simulink model "active_vehicle_controller_functions"  (R2020a)
settings: Solver=ode4  StartTime=0.0  StopTime=inf  FixedStep=1e-3  RelTol=1e-3
InitFcn:
  | clear mex
undefined symbols (not defined in the file or in its folder): DiscIntNeverNeededParam, vicrt_initcallback, vicrt_initmexcallback, vicrt_inputfile, vicrt_simulationmanager
libraries: simulink x1
(part 2 of 6)

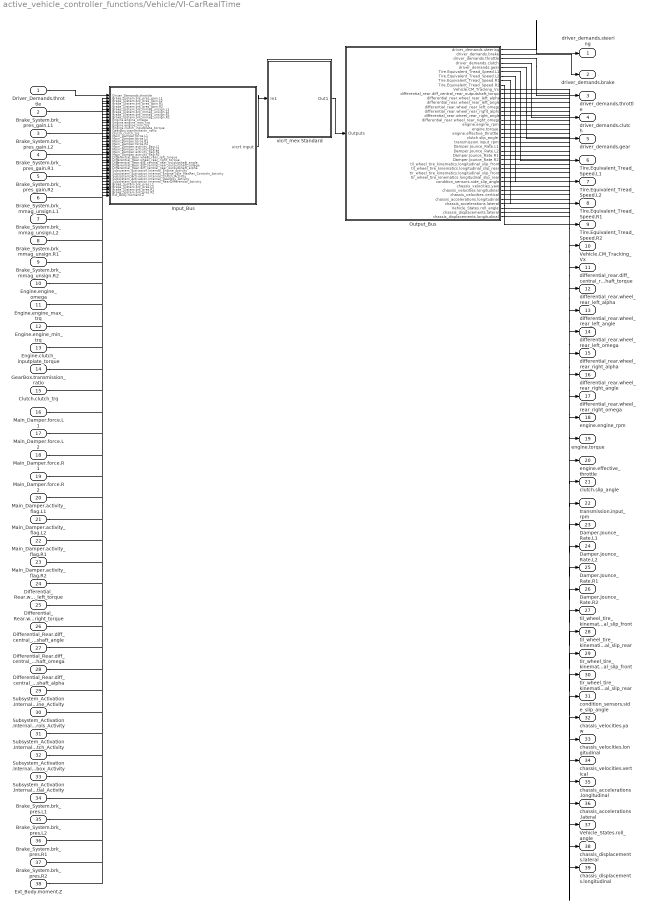
== system active_vehicle_controller_functions/Vehicle/VI-CarRealTime ==
  Driver_Demands.throttle : Inport
  Brake_System.brk_pres_gain.L1 : Inport  Port=2
  Brake_System.brk_pres_gain.L2 : Inport  Port=3
  Brake_System.brk_pres_gain.R1 : Inport  Port=4
  Brake_System.brk_pres_gain.R2 : Inport  Port=5
  Brake_System.brk_mmag_unsign.L1 : Inport  Port=6
  Brake_System.brk_mmag_unsign.L2 : Inport  Port=7
  Brake_System.brk_mmag_unsign.R1 : Inport  Port=8
  Brake_System.brk_mmag_unsign.R2 : Inport  Port=9
  Engine.engine_omega : Inport  Port=10
  Engine.engine_max_trq : Inport  Port=11
  Engine.engine_min_trq : Inport  Port=12
  Engine.clutch_inputplate_torque : Inport  Port=13
  GearBox.transmission_ratio : Inport  Port=14
  Clutch.clutch_trq : Inport  Port=15
  Main_Damper.force.L1 : Inport  Port=16
  Main_Damper.force.L2 : Inport  Port=17
  Main_Damper.force.R1 : Inport  Port=18
  Main_Damper.force.R2 : Inport  Port=19
  Main_Damper.activity_flag.L1 : Inport  Port=20
  Main_Damper.activity_flag.L2 : Inport  Port=21
  Main_Damper.activity_flag.R1 : Inport  Port=22
  Main_Damper.activity_flag.R2 : Inport  Port=23
  Differential_Rear.wheel_rear_left_torque : Inport  Port=24
  Differential_Rear.wheel_rear_right_torque : Inport  Port=25
  Differential_Rear.diff_central_rear_outputshaft_angle : Inport  Port=26
  Differential_Rear.diff_central_rear_outputshaft_omega : Inport  Port=27
  Differential_Rear.diff_central_rear_outputshaft_alpha : Inport  Port=28
  Subsystem_Activation.Internal_Engine_Activity : Inport  Port=29
  Subsystem_Activation.Internal_Engine_Idle_MaxRev_Controls_Activity : Inport  Port=30
  Subsystem_Activation.Internal_Clutch_Activity : Inport  Port=31
  Subsystem_Activation.Internal_Gearbox_Activity : Inport  Port=32
  Subsystem_Activation.Internal_RearDifferential_Activity : Inport  Port=33
  Brake_System.brk_pres.L1 : Inport  Port=34
  Brake_System.brk_pres.L2 : Inport  Port=35
  Brake_System.brk_pres.R1 : Inport  Port=36
  Brake_System.brk_pres.R2 : Inport  Port=37
  Ext_Body.moment.Z : Inport  Port=38
  Input_Bus : Subsystem  LoadFcn=vicrt_initcallback(gcb)
      settings: CopyFcn=vicrt_initcallback(gcb)
  Output_Bus : Subsystem  Description=Outputs
      settings: CopyFcn=set_param(gcb, 'LinkStatus', 'none')
  vicrt_mex Standard : Subsystem  mask{vicrt_inputfile=vicrt_inputfile, vicrt_outprefix='', intStep=0.001, AniFlag=on, inpPortDim=389, outPortDim=1374, NoDirectFeedthrough=on}
      mask prompts: vicrt_inputfile "VI-CarRealtime input file"; vicrt_outprefix "VI-CarRealTime output prefix"; intStep "Integration step"; AniFlag "live animation"; inpPortDim "input port dimension"; outPortDim "output port dimension"; NoDirectFeedthrough "Direct Feedthrough Off"
      mask init:
      | custDriv=[1,1,1];
      settings: CopyFcn=set_param(gcb, 'LinkStatus', 'none')
  driver_demands.steering : Outport  VectorParamsAs1DForOutWhenUnconnected=off
  driver_demands.brake : Outport  Port=2  VectorParamsAs1DForOutWhenUnconnected=off
  driver_demands.throttle : Outport  Port=3  VectorParamsAs1DForOutWhenUnconnected=off
  driver_demands.clutch : Outport  Port=4  VectorParamsAs1DForOutWhenUnconnected=off
  driver_demands.gear : Outport  Port=5  VectorParamsAs1DForOutWhenUnconnected=off
  Tire.Equivalent_Tread_Speed.L1 : Outport  Port=6  VectorParamsAs1DForOutWhenUnconnected=off
  Tire.Equivalent_Tread_Speed.L2 : Outport  Port=7  VectorParamsAs1DForOutWhenUnconnected=off
  Tire.Equivalent_Tread_Speed.R1 : Outport  Port=8  VectorParamsAs1DForOutWhenUnconnected=off
  Tire.Equivalent_Tread_Speed.R2 : Outport  Port=9  VectorParamsAs1DForOutWhenUnconnected=off
  Vehicle.CM_Tracking_Vx : Outport  Port=10  VectorParamsAs1DForOutWhenUnconnected=off
  differential_rear.diff_central_rear_outputshaft_torque : Outport  Port=11  VectorParamsAs1DForOutWhenUnconnected=off
  differential_rear.wheel_rear_left_alpha : Outport  Port=12  VectorParamsAs1DForOutWhenUnconnected=off
  differential_rear.wheel_rear_left_angle : Outport  Port=13  VectorParamsAs1DForOutWhenUnconnected=off
  differential_rear.wheel_rear_left_omega : Outport  Port=14  VectorParamsAs1DForOutWhenUnconnected=off
  differential_rear.wheel_rear_right_alpha : Outport  Port=15  VectorParamsAs1DForOutWhenUnconnected=off
  differential_rear.wheel_rear_right_angle : Outport  Port=16  VectorParamsAs1DForOutWhenUnconnected=off
  differential_rear.wheel_rear_right_omega : Outport  Port=17  VectorParamsAs1DForOutWhenUnconnected=off
  engine.engine_rpm : Outport  Port=18  VectorParamsAs1DForOutWhenUnconnected=off
  engine.torque : Outport  Port=19  VectorParamsAs1DForOutWhenUnconnected=off
  engine.effective_throttle : Outport  Port=20  VectorParamsAs1DForOutWhenUnconnected=off
  clutch.slip_angle : Outport  Port=21  VectorParamsAs1DForOutWhenUnconnected=off
  transmission.input_rpm : Outport  Port=22  VectorParamsAs1DForOutWhenUnconnected=off
  Damper.Jounce_Rate.L1 : Outport  Port=23  VectorParamsAs1DForOutWhenUnconnected=off
  Damper.Jounce_Rate.L2 : Outport  Port=24  VectorParamsAs1DForOutWhenUnconnected=off
  Damper.Jounce_Rate.R1 : Outport  Port=25  VectorParamsAs1DForOutWhenUnconnected=off
  Damper.Jounce_Rate.R2 : Outport  Port=26  VectorParamsAs1DForOutWhenUnconnected=off
  til_wheel_tire_kinematics.longitudinal_slip_front : Outport  Port=27  VectorParamsAs1DForOutWhenUnconnected=off
  til_wheel_tire_kinematics.longitudinal_slip_rear : Outport  Port=28  VectorParamsAs1DForOutWhenUnconnected=off
  tir_wheel_tire_kinematics.longitudinal_slip_front : Outport  Port=29  VectorParamsAs1DForOutWhenUnconnected=off
  tir_wheel_tire_kinematics.longitudinal_slip_rear : Outport  Port=30  VectorParamsAs1DForOutWhenUnconnected=off
  condition_sensors.side_slip_angle : Outport  Port=31  VectorParamsAs1DForOutWhenUnconnected=off
  chassis_velocities.yaw : Outport  Port=32  VectorParamsAs1DForOutWhenUnconnected=off
  chassis_velocities.longitudinal : Outport  Port=33  VectorParamsAs1DForOutWhenUnconnected=off
  chassis_velocities.vertical : Outport  Port=34  VectorParamsAs1DForOutWhenUnconnected=off
  chassis_accelerations.longitudinal : Outport  Port=35  VectorParamsAs1DForOutWhenUnconnected=off
  chassis_accelerations.lateral : Outport  Port=36  VectorParamsAs1DForOutWhenUnconnected=off
  Vehicle_States.roll_angle : Outport  Port=37
  chassis_displacements.lateral : Outport  Port=38
  chassis_displacements.longitudinal : Outport  Port=39
  wires:
  vicrt_mex Standard/1(Out1) -> Output_Bus/1(Outputs)
  Input_Bus/1(vicrt input) -> vicrt_mex Standard/1(In1)
  Driver_Demands.throttle/1 -> Input_Bus/1(Driver_Demands.throttle)
  Brake_System.brk_pres_gain.L1/1 -> Input_Bus/2(Brake_System.brk_pres_gain.L1)
  Brake_System.brk_pres_gain.L2/1 -> Input_Bus/3(Brake_System.brk_pres_gain.L2)
  Brake_System.brk_pres_gain.R1/1 -> Input_Bus/4(Brake_System.brk_pres_gain.R1)
  Brake_System.brk_pres_gain.R2/1 -> Input_Bus/5(Brake_System.brk_pres_gain.R2)
  Brake_System.brk_mmag_unsign.L1/1 -> Input_Bus/6(Brake_System.brk_mmag_unsign.L1)
  Brake_System.brk_mmag_unsign.L2/1 -> Input_Bus/7(Brake_System.brk_mmag_unsign.L2)
  Brake_System.brk_mmag_unsign.R1/1 -> Input_Bus/8(Brake_System.brk_mmag_unsign.R1)
  Brake_System.brk_mmag_unsign.R2/1 -> Input_Bus/9(Brake_System.brk_mmag_unsign.R2)
  Engine.engine_omega/1 -> Input_Bus/10(Engine.engine_omega)
  Engine.engine_max_trq/1 -> Input_Bus/11(Engine.engine_max_trq)
  Engine.engine_min_trq/1 -> Input_Bus/12(Engine.engine_min_trq)
  Engine.clutch_inputplate_torque/1 -> Input_Bus/13(Engine.clutch_inputplate_torque)
  GearBox.transmission_ratio/1 -> Input_Bus/14(GearBox.transmission_ratio)
  Clutch.clutch_trq/1 -> Input_Bus/15(Clutch.clutch_trq)
  Main_Damper.force.L1/1 -> Input_Bus/16(Main_Damper.force.L1)
  Main_Damper.force.L2/1 -> Input_Bus/17(Main_Damper.force.L2)
  Main_Damper.force.R1/1 -> Input_Bus/18(Main_Damper.force.R1)
  Main_Damper.force.R2/1 -> Input_Bus/19(Main_Damper.force.R2)
  Main_Damper.activity_flag.L1/1 -> Input_Bus/20(Main_Damper.activity_flag.L1)
  Main_Damper.activity_flag.L2/1 -> Input_Bus/21(Main_Damper.activity_flag.L2)
  Main_Damper.activity_flag.R1/1 -> Input_Bus/22(Main_Damper.activity_flag.R1)
  Main_Damper.activity_flag.R2/1 -> Input_Bus/23(Main_Damper.activity_flag.R2)
  Differential_Rear.wheel_rear_left_torque/1 -> Input_Bus/24(Differential_Rear.wheel_rear_left_torque)
  Differential_Rear.wheel_rear_right_torque/1 -> Input_Bus/25(Differential_Rear.wheel_rear_right_torque)
  Differential_Rear.diff_central_rear_outputshaft_angle/1 -> Input_Bus/26(Differential_Rear.diff_central_rear_outputshaft_angle)
  Differential_Rear.diff_central_rear_outputshaft_omega/1 -> Input_Bus/27(Differential_Rear.diff_central_rear_outputshaft_omega)
  Differential_Rear.diff_central_rear_outputshaft_alpha/1 -> Input_Bus/28(Differential_Rear.diff_central_rear_outputshaft_alpha)
  Subsystem_Activation.Internal_Engine_Activity/1 -> Input_Bus/29(Subsystem_Activation.Internal_Engine_Activity)
  Subsystem_Activation.Internal_Engine_Idle_MaxRev_Controls_Activity/1 -> Input_Bus/30(Subsystem_Activation.Internal_Engine_Idle_MaxRev_Controls_Activity)
  Subsystem_Activation.Internal_Clutch_Activity/1 -> Input_Bus/31(Subsystem_Activation.Internal_Clutch_Activity)
  Subsystem_Activation.Internal_Gearbox_Activity/1 -> Input_Bus/32(Subsystem_Activation.Internal_Gearbox_Activity)
  Subsystem_Activation.Internal_RearDifferential_Activity/1 -> Input_Bus/33(Subsystem_Activation.Internal_RearDifferential_Activity)
  Brake_System.brk_pres.L1/1 -> Input_Bus/34(Brake_System.brk_pres.L1)
  Brake_System.brk_pres.L2/1 -> Input_Bus/35(Brake_System.brk_pres.L2)
  Brake_System.brk_pres.R1/1 -> Input_Bus/36(Brake_System.brk_pres.R1)
  Brake_System.brk_pres.R2/1 -> Input_Bus/37(Brake_System.brk_pres.R2)
  Ext_Body.moment.Z/1 -> Input_Bus/38(Ext_Body.moment.Z)
  Output_Bus/1(driver_demands.steering) -> driver_demands.steering/1
  Output_Bus/2(driver_demands.brake) -> driver_demands.brake/1
  Output_Bus/3(driver_demands.throttle) -> driver_demands.throttle/1
  Output_Bus/4(driver_demands.clutch) -> driver_demands.clutch/1
  Output_Bus/5(driver_demands.gear) -> driver_demands.gear/1
  Output_Bus/6(Tire.Equivalent_Tread_Speed.L1) -> Tire.Equivalent_Tread_Speed.L1/1
  Output_Bus/7(Tire.Equivalent_Tread_Speed.L2) -> Tire.Equivalent_Tread_Speed.L2/1
  Output_Bus/8(Tire.Equivalent_Tread_Speed.R1) -> Tire.Equivalent_Tread_Speed.R1/1
  Output_Bus/9(Tire.Equivalent_Tread_Speed.R2) -> Tire.Equivalent_Tread_Speed.R2/1
  Output_Bus/10(Vehicle.CM_Tracking_Vx) -> Vehicle.CM_Tracking_Vx/1
  Output_Bus/11(differential_rear.diff_central_rear_outputshaft_torque) -> differential_rear.diff_central_rear_outputshaft_torque/1
  Output_Bus/12(differential_rear.wheel_rear_left_alpha) -> differential_rear.wheel_rear_left_alpha/1
  Output_Bus/13(differential_rear.wheel_rear_left_angle) -> differential_rear.wheel_rear_left_angle/1
  Output_Bus/14(differential_rear.wheel_rear_left_omega) -> differential_rear.wheel_rear_left_omega/1
  Output_Bus/15(differential_rear.wheel_rear_right_alpha) -> differential_rear.wheel_rear_right_alpha/1
  Output_Bus/16(differential_rear.wheel_rear_right_angle) -> differential_rear.wheel_rear_right_angle/1
  Output_Bus/17(differential_rear.wheel_rear_right_omega) -> differential_rear.wheel_rear_right_omega/1
  Output_Bus/18(engine.engine_rpm) -> engine.engine_rpm/1
  Output_Bus/19(engine.torque) -> engine.torque/1
  Output_Bus/20(engine.effective_throttle) -> engine.effective_throttle/1
  Output_Bus/21(clutch.slip_angle) -> clutch.slip_angle/1
  Output_Bus/22(transmission.input_rpm) -> transmission.input_rpm/1
  Output_Bus/23(Damper.Jounce_Rate.L1) -> Damper.Jounce_Rate.L1/1
  Output_Bus/24(Damper.Jounce_Rate.L2) -> Damper.Jounce_Rate.L2/1
  Output_Bus/25(Damper.Jounce_Rate.R1) -> Damper.Jounce_Rate.R1/1
  Output_Bus/26(Damper.Jounce_Rate.R2) -> Damper.Jounce_Rate.R2/1
  Output_Bus/27(til_wheel_tire_kinematics.longitudinal_slip_front) -> til_wheel_tire_kinematics.longitudinal_slip_front/1
  Output_Bus/28(til_wheel_tire_kinematics.longitudinal_slip_rear) -> til_wheel_tire_kinematics.longitudinal_slip_rear/1
  Output_Bus/29(tir_wheel_tire_kinematics.longitudinal_slip_front) -> tir_wheel_tire_kinematics.longitudinal_slip_front/1
  Output_Bus/30(tir_wheel_tire_kinematics.longitudinal_slip_rear) -> tir_wheel_tire_kinematics.longitudinal_slip_rear/1
  Output_Bus/31(condition_sensors.side_slip_angle) -> condition_sensors.side_slip_angle/1
  Output_Bus/32(chassis_velocities.yaw) -> chassis_velocities.yaw/1
  Output_Bus/33(chassis_velocities.longitudinal) -> chassis_velocities.longitudinal/1
  Output_Bus/34(chassis_velocities.vertical) -> chassis_velocities.vertical/1
  Output_Bus/35(chassis_accelerations.longitudinal) -> chassis_accelerations.longitudinal/1
  Output_Bus/36(chassis_accelerations.lateral) -> chassis_accelerations.lateral/1
  Output_Bus/37(Vehicle_States.roll_angle) -> Vehicle_States.roll_angle/1
  Output_Bus/38(chassis_displacements.lateral) -> chassis_displacements.lateral/1
  Output_Bus/39(chassis_displacements.longitudinal) -> chassis_displacements.longitudinal/1

== system active_vehicle_controller_functions/Driveline/Clutch/lag ==
  In1 : Inport
  Memory5 : Memory  InheritSampleTime=on
  Sum : Sum  Inputs=|++  OutDataTypeStr=Inherit: Same as first input
  "gain_1 " : Gain  Gain=1-exp(-2*pi*0.001)  OutDataTypeStr=Inherit: Same as input  ParamDataTypeStr=Inherit: Same as input
  gain_1 1 : Gain  Gain=exp(-2*pi*0.001)  OutDataTypeStr=Inherit: Same as input  ParamDataTypeStr=Inherit: Same as input
  Out1 : Outport  VectorParamsAs1DForOutWhenUnconnected=off
  wires:
  In1/1 -> "gain_1 "/1
  "gain_1 "/1 -> Sum/1
  Sum/1 -> Memory5/1, Out1/1
  Memory5/1 -> gain_1 1/1
  gain_1 1/1 -> Sum/2

== system active_vehicle_controller_functions/Driveline/Engine/Engine Maps ==
  RPM : Inport
  Throttle : Inport  Port=2
  0-throttle : Constant  Value=0
  Demux : Demux  Outputs=3
  Engine Torque : Lookup2D  RowIndex=|  ColumnIndex=[0,1]  Table="[0.0  0.0; -20.0  120.0;-42.0  270.0; -44.0  400.0;-46.0  490.0; -48.0  526.0;-50.0  620.0; -50.0  716.0;-50.0  808.0; -50.0  910.0; -50.0  950.0; -50.0  970.0;-50.0  936.0; -50.0  924.0; -52.0  910.0; -56.0  854.0; -60.0  740.0; -64.0  690.0; -68.0  650.0;]"
      | [0.0	
      | 500.0	
      | 1000.0	
      | 1500.0	
      | 2000.0	
      | 2500.0	
      | 3000.0	
      | 3500.0	
      | 4000.0	
      | 4500.0	
      | 5000.0	
      | 5500.0	
      | 6000.0	
      | 6250.0	
      | 6500.0	
      | 6750.0	
      | 7000.0	
      | 7500.0	
      | 8000.0]
  FullThrottle : Constant
  Memory1 : Memory
  Mux : Mux  Inputs=3
  Rpm control : Subsystem
  Saturation Dynamic : simulink/Discontinuities/Saturation Dynamic  OutMin=[]  OutMax=[]  OutDataTypeStr=Inherit: Same as second input  OutDataType=sfix(16)  OutScaling=2^-10  DoSatur=off
  Switch : Switch  Criteria=u2 > Threshold
  Zero : Constant  Value=[0,0,0]
  rpm2rad_sec : Gain  Gain=(60/2/pi)^-1  OutDataTypeStr=Inherit: Same as input  ParamDataTypeStr=Inherit: Same as input
  scale : Gain  Gain=0.01  OutDataTypeStr=Inherit: Same as input  ParamDataTypeStr=Inherit: Same as input
  MaxEngineTorque : Outport  VectorParamsAs1DForOutWhenUnconnected=off
  MinEngineTorque : Outport  Port=2  VectorParamsAs1DForOutWhenUnconnected=off
  EngineTorque : Outport  Port=3  VectorParamsAs1DForOutWhenUnconnected=off
  wires:
  Throttle/1 -> Rpm control/2(Throttle)
  scale/1 -> Mux/2
  FullThrottle/1 -> Mux/1
  Mux/1 -> Engine Torque/2
  RPM/1 -> Engine Torque/1, rpm2rad_sec/1
  Demux/1 -> MaxEngineTorque/1, Saturation Dynamic/1
  Demux/3 -> MinEngineTorque/1, Saturation Dynamic/3
  rpm2rad_sec/1 -> Rpm control/1(engine omega)
  0-throttle/1 -> Mux/3
  Rpm control/1(Throttle mod) -> scale/1
  Saturation Dynamic/1 -> EngineTorque/1
  Demux/2 -> Saturation Dynamic/2
  [InternalEngineActive] -> Switch/2
  Zero/1 -> Switch/1
  Switch/1 -> Demux/1
  Memory1/1 -> Switch/3
  Engine Torque/1 -> Memory1/1

== system active_vehicle_controller_functions/Driveline/Engine/ThrottleOff (from ESP) ==
  Constant : Constant
  Sum : Sum  Inputs=|+-  OutDataTypeStr=Inherit: Same as first input
  ThrottleOffGain1 : Gain  Gain=1-ThrottleOffScale  OutDataTypeStr=Inherit: Same as input  ParamDataTypeStr=Inherit: Same as input
  Transfer Fcn : TransferFcn  Denominator="[0.02  1]"
  ThrottleGain : Outport  VectorParamsAs1DForOutWhenUnconnected=off
  wires:
  ThrottleOffGain1/1 -> Transfer Fcn/1
  Constant/1 -> Sum/1
  Transfer Fcn/1 -> Sum/2
  [ThrottleOff] -> ThrottleOffGain1/1
  Sum/1 -> ThrottleGain/1

== system active_vehicle_controller_functions/Driveline/Rear Differential/Limited Slip Diff ==
  diff center front output shaft torque : Inport
  wheel front right omega : Inport  Port=2
  wheel front left omega : Inport  Port=3
  " " : Memory
  "   " : Memory
  "    " : Memory
  "       " : Memory
  "          " : Math  Operator=pow  SignedPower=on  SaturateOnIntegerOverflow=on
  AbsDeltaOmega : Abs
  AbsT : Abs
  C0 : Constant  Value=C0
  C1 : Gain  Gain=C1
  C2 : Gain  Gain=C2
  C3 : Constant  Value=C3
  C4 : Gain  Gain=-1
  DeltaTorqueL : Product  Inputs=**
  DeltaTorqueR : Product  Inputs=**
  Sign : Lookup  InputValues=[-1000 -100 -1 -0.5 0 .5 1 100 1000]  Table=[-1 -1 -1 0 0 0 1 1 1]
  Sum : Sum  Inputs=+-
  Sum3 : Sum  Inputs=+++  SaturateOnIntegerOverflow=on
  wheel front left torque : Outport  VectorParamsAs1DForOutWhenUnconnected=off
  wheel front right torque : Outport  Port=2  VectorParamsAs1DForOutWhenUnconnected=off
  wires:
  C0/1 -> Sum3/1
  C2/1 -> "          "/1
  "    "/1 -> DeltaTorqueL/2, DeltaTorqueR/2
  "       "/1 -> Sum3/3
  DeltaTorqueR/1 -> C4/1
  Sign/1 -> "    "/1
  C1/1 -> Sum3/2
  Sum3/1 -> DeltaTorqueR/1, DeltaTorqueL/1
  C4/1 -> wheel front right torque/1
  AbsT/1 -> "   "/1
  "          "/1 -> "       "/1
  AbsDeltaOmega/1 -> " "/1
  wheel front left omega/1 -> Sum/2
  "   "/1 -> C1/1
  diff center front output shaft torque/1 -> AbsT/1
  " "/1 -> C2/1
  DeltaTorqueL/1 -> wheel front left torque/1
  C3/1 -> "          "/2
  Sum/1 -> Sign/1, AbsDeltaOmega/1
  wheel front right omega/1 -> Sum/1

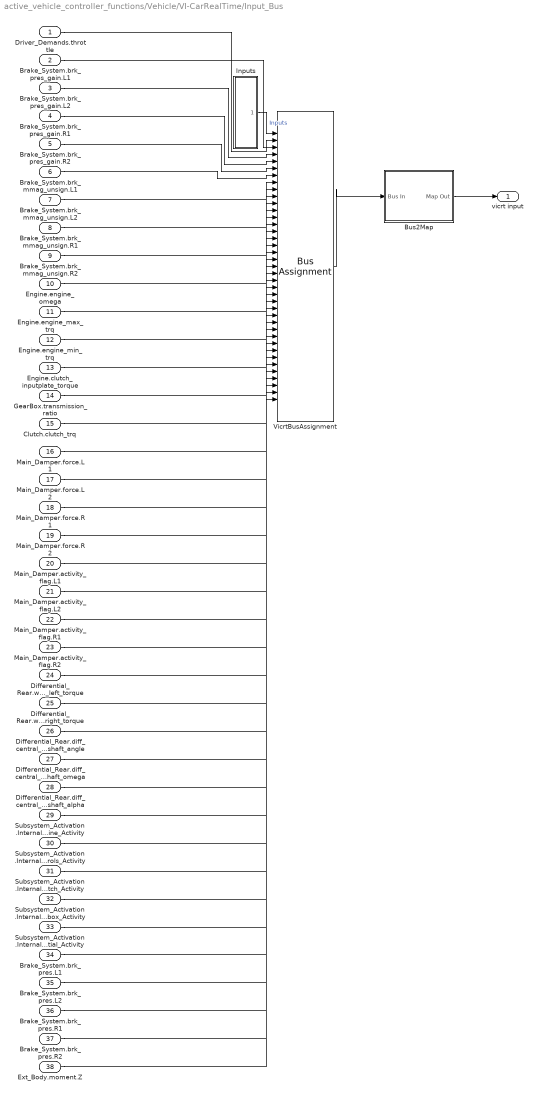
== system active_vehicle_controller_functions/Vehicle/VI-CarRealTime/Input_Bus ==
  Driver_Demands.throttle : Inport
  Brake_System.brk_pres_gain.L1 : Inport  Port=2
  Brake_System.brk_pres_gain.L2 : Inport  Port=3
  Brake_System.brk_pres_gain.R1 : Inport  Port=4
  Brake_System.brk_pres_gain.R2 : Inport  Port=5
  Brake_System.brk_mmag_unsign.L1 : Inport  Port=6
  Brake_System.brk_mmag_unsign.L2 : Inport  Port=7
  Brake_System.brk_mmag_unsign.R1 : Inport  Port=8
  Brake_System.brk_mmag_unsign.R2 : Inport  Port=9
  Engine.engine_omega : Inport  Port=10
  Engine.engine_max_trq : Inport  Port=11
  Engine.engine_min_trq : Inport  Port=12
  Engine.clutch_inputplate_torque : Inport  Port=13
  GearBox.transmission_ratio : Inport  Port=14
  Clutch.clutch_trq : Inport  Port=15
  Main_Damper.force.L1 : Inport  Port=16
  Main_Damper.force.L2 : Inport  Port=17
  Main_Damper.force.R1 : Inport  Port=18
  Main_Damper.force.R2 : Inport  Port=19
  Main_Damper.activity_flag.L1 : Inport  Port=20
  Main_Damper.activity_flag.L2 : Inport  Port=21
  Main_Damper.activity_flag.R1 : Inport  Port=22
  Main_Damper.activity_flag.R2 : Inport  Port=23
  Differential_Rear.wheel_rear_left_torque : Inport  Port=24
  Differential_Rear.wheel_rear_right_torque : Inport  Port=25
  Differential_Rear.diff_central_rear_outputshaft_angle : Inport  Port=26
  Differential_Rear.diff_central_rear_outputshaft_omega : Inport  Port=27
  Differential_Rear.diff_central_rear_outputshaft_alpha : Inport  Port=28
  Subsystem_Activation.Internal_Engine_Activity : Inport  Port=29
  Subsystem_Activation.Internal_Engine_Idle_MaxRev_Controls_Activity : Inport  Port=30
  Subsystem_Activation.Internal_Clutch_Activity : Inport  Port=31
  Subsystem_Activation.Internal_Gearbox_Activity : Inport  Port=32
  Subsystem_Activation.Internal_RearDifferential_Activity : Inport  Port=33
  Brake_System.brk_pres.L1 : Inport  Port=34
  Brake_System.brk_pres.L2 : Inport  Port=35
  Brake_System.brk_pres.R1 : Inport  Port=36
  Brake_System.brk_pres.R2 : Inport  Port=37
  Ext_Body.moment.Z : Inport  Port=38
  Bus2Map : Subsystem
  Inputs : Subsystem
  VicrtBusAssignment : BusAssignment  AssignedSignals=Driver_Demands.throttle,Brake_System.brk_pres_gain.L1,Brake_System.brk_pres_gain.L2,Brake_System.brk_pres_gain.R1,Brake_System.brk_pres_gain.R2,Brake_System.brk_mmag_unsign.L1,Brake_System.brk_mmag_unsign.L2,Brake_System.brk_mmag_unsign.R1,Brake_System.brk_mmag_unsign.R2,Engine.engine_omega,Engine.engine_max_trq,Engine.engine_min_trq,Engine.clutch_inputplate_torque,GearBox.transmission_ratio,Clutch.clutch_trq,Main_Damper.force.L1,Main_Damper.force.L2,Main_Damper.force.R1,Main_Damper.force.R2,Main_Damper.activity_flag.L1,Main_Damper.activity_flag.L2,Main_Damper.activity_flag.R1,Main_Damper.activity_flag.R2,Differential_Rear.wheel_rear_left_torque,Differential_Rear.wheel_rear_right_torque,Differential_Rear.diff_central_rear_outputshaft_angle,Differential_Rear.diff_central_rear_outputshaft_omega,Differential_Rear.diff_central_rear_outputshaft_alpha,Subsystem_Activation.Internal_Engine_Activity,Subsystem_Activation.Internal_Engine_Idle_MaxRev_Controls_Activity,Subsystem_Activation.Internal_Clutch_Activity,Subsystem_Activation.Internal_Gearbox_Activity,Subsystem_Activation.Internal_RearDifferential_Activity,Brake_System.brk_pres.L1,Brake_System.brk_pres.L2,Brake_System.brk_pres.R1,Brake_System.brk_pres.R2,Ext_Body.moment.Z
  vicrt input : Outport  VectorParamsAs1DForOutWhenUnconnected=off
  wires:
  Bus2Map/1(Map Out) -> vicrt input/1
  VicrtBusAssignment/1 -> Bus2Map/1(Bus In)
  Inputs/1(Inputs) -> VicrtBusAssignment/1  "Inputs"
  Driver_Demands.throttle/1 -> VicrtBusAssignment/2
  Brake_System.brk_pres_gain.L1/1 -> VicrtBusAssignment/3
  Brake_System.brk_pres_gain.L2/1 -> VicrtBusAssignment/4
  Brake_System.brk_pres_gain.R1/1 -> VicrtBusAssignment/5
  Brake_System.brk_pres_gain.R2/1 -> VicrtBusAssignment/6
  Brake_System.brk_mmag_unsign.L1/1 -> VicrtBusAssignment/7
  Brake_System.brk_mmag_unsign.L2/1 -> VicrtBusAssignment/8
  Brake_System.brk_mmag_unsign.R1/1 -> VicrtBusAssignment/9
  Brake_System.brk_mmag_unsign.R2/1 -> VicrtBusAssignment/10
  Engine.engine_omega/1 -> VicrtBusAssignment/11
  Engine.engine_max_trq/1 -> VicrtBusAssignment/12
  Engine.engine_min_trq/1 -> VicrtBusAssignment/13
  Engine.clutch_inputplate_torque/1 -> VicrtBusAssignment/14
  GearBox.transmission_ratio/1 -> VicrtBusAssignment/15
  Clutch.clutch_trq/1 -> VicrtBusAssignment/16
  Main_Damper.force.L1/1 -> VicrtBusAssignment/17
  Main_Damper.force.L2/1 -> VicrtBusAssignment/18
  Main_Damper.force.R1/1 -> VicrtBusAssignment/19
  Main_Damper.force.R2/1 -> VicrtBusAssignment/20
  Main_Damper.activity_flag.L1/1 -> VicrtBusAssignment/21
  Main_Damper.activity_flag.L2/1 -> VicrtBusAssignment/22
  Main_Damper.activity_flag.R1/1 -> VicrtBusAssignment/23
  Main_Damper.activity_flag.R2/1 -> VicrtBusAssignment/24
  Differential_Rear.wheel_rear_left_torque/1 -> VicrtBusAssignment/25
  Differential_Rear.wheel_rear_right_torque/1 -> VicrtBusAssignment/26
  Differential_Rear.diff_central_rear_outputshaft_angle/1 -> VicrtBusAssignment/27
  Differential_Rear.diff_central_rear_outputshaft_omega/1 -> VicrtBusAssignment/28
  Differential_Rear.diff_central_rear_outputshaft_alpha/1 -> VicrtBusAssignment/29
  Subsystem_Activation.Internal_Engine_Activity/1 -> VicrtBusAssignment/30
  Subsystem_Activation.Internal_Engine_Idle_MaxRev_Controls_Activity/1 -> VicrtBusAssignment/31
  Subsystem_Activation.Internal_Clutch_Activity/1 -> VicrtBusAssignment/32
  Subsystem_Activation.Internal_Gearbox_Activity/1 -> VicrtBusAssignment/33
  Subsystem_Activation.Internal_RearDifferential_Activity/1 -> VicrtBusAssignment/34
  Brake_System.brk_pres.L1/1 -> VicrtBusAssignment/35
  Brake_System.brk_pres.L2/1 -> VicrtBusAssignment/36
  Brake_System.brk_pres.R1/1 -> VicrtBusAssignment/37
  Brake_System.brk_pres.R2/1 -> VicrtBusAssignment/38
  Ext_Body.moment.Z/1 -> VicrtBusAssignment/39

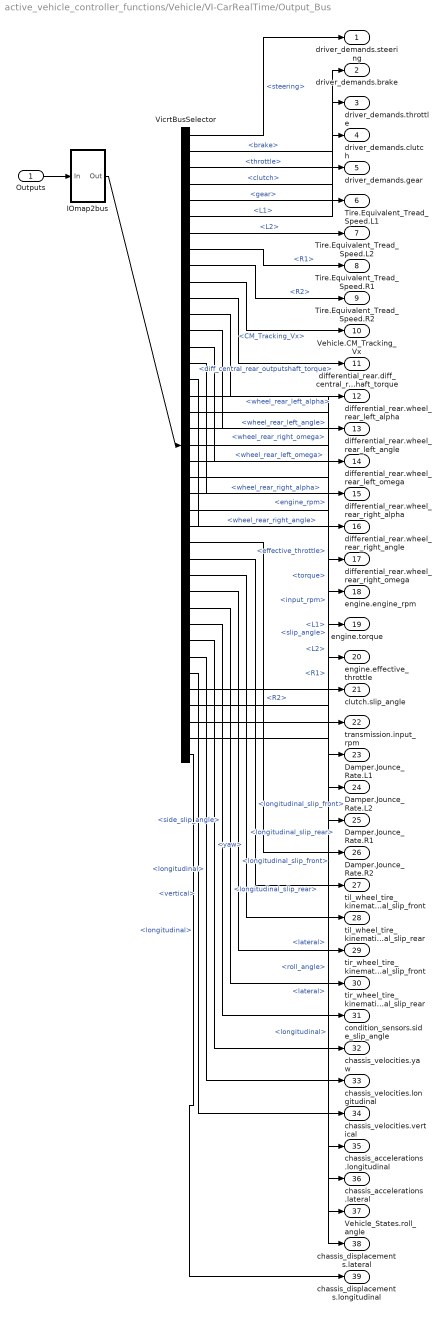
== system active_vehicle_controller_functions/Vehicle/VI-CarRealTime/Output_Bus ==
  Outputs : Inport
  IOmap2bus : Subsystem
  VicrtBusSelector : BusSelector  OutputSignals=driver_demands.steering,driver_demands.brake,driver_demands.throttle,driver_demands.clutch,driver_demands.gear,Tire.Equivalent_Tread_Speed.L1,Tire.Equivalent_Tread_Speed.L2,Tire.Equivalent_Tread_Speed.R1,Tire.Equivalent_Tread_Speed.R2,Vehicle.CM_Tracking_Vx,differential_rear.diff_central_rear_outputshaft_torque,differential_rear.wheel_rear_left_alpha,differential_rear.wheel_rear_left_angle,differential_rear.wheel_rear_left_omega,differential_rear.wheel_rear_right_alpha,differential_rear.wheel_rear_right_angle,differential_rear.wheel_rear_right_omega,engine.engine_rpm,engine.torque,engine.effective_throttle,clutch.slip_angle,transmission.input_rpm,Damper.Jounce_Rate.L1,Damper.Jounce_Rate.L2,Damper.Jounce_Rate.R1,Damper.Jounce_Rate.R2,til_wheel_tire_kinematics.longitudinal_slip_front,til_wheel_tire_kinematics.longitudinal_slip_rear,tir_wheel_tire_kinematics.longitudinal_slip_front,tir_wheel_tire_kinematics.longitudinal_slip_rear,condition_sensors.side_slip_angle,chassis_velocities.yaw,chassis_velocities.longitudinal,chassis_velocities.vertical,chassis_accelerations.longitudinal,chassis_accelerations.lateral,Vehicle_States.roll_angle,chassis_displacements.lateral,chassis_displacements.longitudinal
  driver_demands.steering : Outport  VectorParamsAs1DForOutWhenUnconnected=off
  driver_demands.brake : Outport  Port=2  VectorParamsAs1DForOutWhenUnconnected=off
  driver_demands.throttle : Outport  Port=3  VectorParamsAs1DForOutWhenUnconnected=off
  driver_demands.clutch : Outport  Port=4  VectorParamsAs1DForOutWhenUnconnected=off
  driver_demands.gear : Outport  Port=5  VectorParamsAs1DForOutWhenUnconnected=off
  Tire.Equivalent_Tread_Speed.L1 : Outport  Port=6  VectorParamsAs1DForOutWhenUnconnected=off
  Tire.Equivalent_Tread_Speed.L2 : Outport  Port=7  VectorParamsAs1DForOutWhenUnconnected=off
  Tire.Equivalent_Tread_Speed.R1 : Outport  Port=8  VectorParamsAs1DForOutWhenUnconnected=off
  Tire.Equivalent_Tread_Speed.R2 : Outport  Port=9  VectorParamsAs1DForOutWhenUnconnected=off
  Vehicle.CM_Tracking_Vx : Outport  Port=10  VectorParamsAs1DForOutWhenUnconnected=off
  differential_rear.diff_central_rear_outputshaft_torque : Outport  Port=11  VectorParamsAs1DForOutWhenUnconnected=off
  differential_rear.wheel_rear_left_alpha : Outport  Port=12  VectorParamsAs1DForOutWhenUnconnected=off
  differential_rear.wheel_rear_left_angle : Outport  Port=13  VectorParamsAs1DForOutWhenUnconnected=off
  differential_rear.wheel_rear_left_omega : Outport  Port=14  VectorParamsAs1DForOutWhenUnconnected=off
  differential_rear.wheel_rear_right_alpha : Outport  Port=15  VectorParamsAs1DForOutWhenUnconnected=off
  differential_rear.wheel_rear_right_angle : Outport  Port=16  VectorParamsAs1DForOutWhenUnconnected=off
  differential_rear.wheel_rear_right_omega : Outport  Port=17  VectorParamsAs1DForOutWhenUnconnected=off
  engine.engine_rpm : Outport  Port=18  VectorParamsAs1DForOutWhenUnconnected=off
  engine.torque : Outport  Port=19  VectorParamsAs1DForOutWhenUnconnected=off
  engine.effective_throttle : Outport  Port=20  VectorParamsAs1DForOutWhenUnconnected=off
  clutch.slip_angle : Outport  Port=21  VectorParamsAs1DForOutWhenUnconnected=off
  transmission.input_rpm : Outport  Port=22  VectorParamsAs1DForOutWhenUnconnected=off
  Damper.Jounce_Rate.L1 : Outport  Port=23  VectorParamsAs1DForOutWhenUnconnected=off
  Damper.Jounce_Rate.L2 : Outport  Port=24  VectorParamsAs1DForOutWhenUnconnected=off
  Damper.Jounce_Rate.R1 : Outport  Port=25  VectorParamsAs1DForOutWhenUnconnected=off
  Damper.Jounce_Rate.R2 : Outport  Port=26  VectorParamsAs1DForOutWhenUnconnected=off
  til_wheel_tire_kinematics.longitudinal_slip_front : Outport  Port=27  VectorParamsAs1DForOutWhenUnconnected=off
  til_wheel_tire_kinematics.longitudinal_slip_rear : Outport  Port=28  VectorParamsAs1DForOutWhenUnconnected=off
  tir_wheel_tire_kinematics.longitudinal_slip_front : Outport  Port=29  VectorParamsAs1DForOutWhenUnconnected=off
  tir_wheel_tire_kinematics.longitudinal_slip_rear : Outport  Port=30  VectorParamsAs1DForOutWhenUnconnected=off
  condition_sensors.side_slip_angle : Outport  Port=31  VectorParamsAs1DForOutWhenUnconnected=off
  chassis_velocities.yaw : Outport  Port=32  VectorParamsAs1DForOutWhenUnconnected=off
  chassis_velocities.longitudinal : Outport  Port=33  VectorParamsAs1DForOutWhenUnconnected=off
  chassis_velocities.vertical : Outport  Port=34  VectorParamsAs1DForOutWhenUnconnected=off
  chassis_accelerations.longitudinal : Outport  Port=35  VectorParamsAs1DForOutWhenUnconnected=off
  chassis_accelerations.lateral : Outport  Port=36  VectorParamsAs1DForOutWhenUnconnected=off
  Vehicle_States.roll_angle : Outport  Port=37
  chassis_displacements.lateral : Outport  Port=38
  chassis_displacements.longitudinal : Outport  Port=39
  wires:
  IOmap2bus/1(Out) -> VicrtBusSelector/1
  Outputs/1 -> IOmap2bus/1(In)
  VicrtBusSelector/1 -> driver_demands.steering/1  "<steering>"
  VicrtBusSelector/2 -> driver_demands.brake/1  "<brake>"
  VicrtBusSelector/3 -> driver_demands.throttle/1  "<throttle>"
  VicrtBusSelector/4 -> driver_demands.clutch/1  "<clutch>"
  VicrtBusSelector/5 -> driver_demands.gear/1  "<gear>"
  VicrtBusSelector/6 -> Tire.Equivalent_Tread_Speed.L1/1  "<L1>"
  VicrtBusSelector/7 -> Tire.Equivalent_Tread_Speed.L2/1  "<L2>"
  VicrtBusSelector/8 -> Tire.Equivalent_Tread_Speed.R1/1  "<R1>"
  VicrtBusSelector/9 -> Tire.Equivalent_Tread_Speed.R2/1  "<R2>"
  VicrtBusSelector/10 -> Vehicle.CM_Tracking_Vx/1  "<CM_Tracking_Vx>"
  VicrtBusSelector/11 -> differential_rear.diff_central_rear_outputshaft_torque/1  "<diff_central_rear_outputshaft_torque>"
  VicrtBusSelector/12 -> differential_rear.wheel_rear_left_alpha/1  "<wheel_rear_left_alpha>"
  VicrtBusSelector/13 -> differential_rear.wheel_rear_left_angle/1  "<wheel_rear_left_angle>"
  VicrtBusSelector/14 -> differential_rear.wheel_rear_left_omega/1  "<wheel_rear_left_omega>"
  VicrtBusSelector/15 -> differential_rear.wheel_rear_right_alpha/1  "<wheel_rear_right_alpha>"
  VicrtBusSelector/16 -> differential_rear.wheel_rear_right_angle/1  "<wheel_rear_right_angle>"
  VicrtBusSelector/17 -> differential_rear.wheel_rear_right_omega/1  "<wheel_rear_right_omega>"
  VicrtBusSelector/18 -> engine.engine_rpm/1  "<engine_rpm>"
  VicrtBusSelector/19 -> engine.torque/1  "<torque>"
  VicrtBusSelector/20 -> engine.effective_throttle/1  "<effective_throttle>"
  VicrtBusSelector/21 -> clutch.slip_angle/1  "<slip_angle>"
  VicrtBusSelector/22 -> transmission.input_rpm/1  "<input_rpm>"
  VicrtBusSelector/23 -> Damper.Jounce_Rate.L1/1  "<L1>"
  VicrtBusSelector/24 -> Damper.Jounce_Rate.L2/1  "<L2>"
  VicrtBusSelector/25 -> Damper.Jounce_Rate.R1/1  "<R1>"
  VicrtBusSelector/26 -> Damper.Jounce_Rate.R2/1  "<R2>"
  VicrtBusSelector/27 -> til_wheel_tire_kinematics.longitudinal_slip_front/1  "<longitudinal_slip_front>"
  VicrtBusSelector/28 -> til_wheel_tire_kinematics.longitudinal_slip_rear/1  "<longitudinal_slip_rear>"
  VicrtBusSelector/29 -> tir_wheel_tire_kinematics.longitudinal_slip_front/1  "<longitudinal_slip_front>"
  VicrtBusSelector/30 -> tir_wheel_tire_kinematics.longitudinal_slip_rear/1  "<longitudinal_slip_rear>"
  VicrtBusSelector/31 -> condition_sensors.side_slip_angle/1  "<side_slip_angle>"
  VicrtBusSelector/32 -> chassis_velocities.yaw/1  "<yaw>"
  VicrtBusSelector/33 -> chassis_velocities.longitudinal/1  "<longitudinal>"
  VicrtBusSelector/34 -> chassis_velocities.vertical/1  "<vertical>"
  VicrtBusSelector/35 -> chassis_accelerations.longitudinal/1  "<longitudinal>"
  VicrtBusSelector/36 -> chassis_accelerations.lateral/1  "<lateral>"
  VicrtBusSelector/37 -> Vehicle_States.roll_angle/1  "<roll_angle>"
  VicrtBusSelector/38 -> chassis_displacements.lateral/1  "<lateral>"
  VicrtBusSelector/39 -> chassis_displacements.longitudinal/1  "<longitudinal>"

== system active_vehicle_controller_functions/Vehicle/VI-CarRealTime/vicrt_mex Standard ==
  In1 : Inport
  vicrt_mex : S-Function  InitFcn=vicrt_initmexcallback(gcb);  FunctionName=vicrt_mex  Parameters=vicrt_inputfile,vicrt_outprefix,AniFlag,intStep,inpPortDim,outPortDim,NoDirectFeedthrough  SFunctionDeploymentMode=off  EnableBusSupport=off
  Out1 : Outport  VectorParamsAs1DForOutWhenUnconnected=off
  wires:
  In1/1 -> vicrt_mex/1
  vicrt_mex/1 -> Out1/1

== system active_vehicle_controller_functions/Driveline/Engine/Engine Maps/Rpm control ==
  engine omega : Inport
  Throttle : Inport  Port=2
  Add : Sum  OutDataTypeStr=Inherit: Same as first input
  Add1 : Sum  OutDataTypeStr=Inherit: Same as first input
  Embedded MATLAB Function : MATLAB Function  TreatAsAtomicUnit=on
  MinMax : MinMax  Function=max  Inputs=2
  MinMax1 : MinMax  Inputs=2
  MinMax2 : MinMax  Function=max  Inputs=2
  Product : Product  RndMeth=Zero  OutDataTypeStr=Inherit: Same as first input
  full throttle : Constant  Value=100
  idle control : Subsystem
  idle speed : Constant  Value=3000
  rpm2rad_sec : Gain  Gain=(60/2/pi)^-1  OutDataTypeStr=Inherit: Same as input  ParamDataTypeStr=Inherit: Same as input
  rpm2rad_sec1 : Gain  Gain=(60/2/pi)^-1  OutDataTypeStr=Inherit: Same as input  ParamDataTypeStr=Inherit: Same as input
  rpm2rad_sec2 : Gain  Gain=(60/2/pi)^-1  OutDataTypeStr=Inherit: Same as input  ParamDataTypeStr=Inherit: Same as input
  saturation RPM : Constant  Value=100
  upper engine limit RPM : Constant  Value=8000
  zero : Constant  Value=0
  Throttle mod : Outport  VectorParamsAs1DForOutWhenUnconnected=off
  wires:
  zero/1 -> MinMax/1, MinMax2/1
  engine omega/1 -> MinMax/2, idle control/1(engine omega)
  upper engine limit RPM/1 -> Add/1, rpm2rad_sec/1
  saturation RPM/1 -> Add/2
  Add/1 -> rpm2rad_sec1/1
  rpm2rad_sec/1 -> Embedded MATLAB Function/2(x1)
  rpm2rad_sec1/1 -> Embedded MATLAB Function/3(x2)
  idle speed/1 -> rpm2rad_sec2/1
  rpm2rad_sec2/1 -> idle control/2(idle speed)
  idle control/1(rpm_idle_contrlol) -> Add1/2
  full throttle/1 -> MinMax1/1
  Throttle/1 -> MinMax1/2
  MinMax1/1 -> Product/2
  Product/1 -> MinMax2/2
  MinMax2/1 -> Add1/1
  Add1/1 -> Throttle mod/1
  MinMax/1 -> Embedded MATLAB Function/1(x)
  Embedded MATLAB Function/1(thr) -> Product/1
